simulink model "PosAvail"  (R2018b)
settings: Solver=FixedStepDiscrete  StartTime=0.0  StopTime=10.0  FixedStep=0.01  RelTol=1e-3
settings Model: Creator=su3dcu  LastModifiedBy=su3dcu
settings DataIOCC: SaveFormat=StructureWithTime  ReturnWorkspaceOutputs=on
settings OptimizationCC: DefaultParameterBehavior=Inlined  EnhancedBackFolding=on  PassReuseOutputArgsAs=Individual arguments  ZeroExternalMemoryAtStartup=off  ZeroInternalMemoryAtStartup=off  OptimizeBlockOrder=speed  DifferentSizesBufferReuse=on  OptimizationCustomize=off
settings DebuggingCC: ParameterTunabilityLossMsg=error
settings HardwareCC: ProdBitPerPointer=32  ProdBitPerSizeT=32  ProdBitPerPtrDiffT=32  ProdLargestAtomicFloat=None  ProdWordSize=32  ProdHWDeviceType=Renesas->RH850
settings ModelReferenceCC: ModelReferenceNumInstancesAllowed=Single
settings SFSimCC: SimCustomHeaderCode="#include\"Rte_Type.h\""  MATLABDynamicMemAlloc=off
settings RTWCC: SystemTargetFile=autosar.tlc  GenCodeOnly=on  TemplateMakefile=ert_default_tmf  Description=AUTOSAR  GenerateReport=on  IncludeHyperlinkInReport=on  LaunchReport=on  CodeExecutionProfiling=on  GenerateTraceInfo=on  GenerateTraceReport=on  GenerateTraceReportSl=on  GenerateTraceReportSf=on  GenerateTraceReportEml=on  GenerateCodeMetricsReport=on
settings CodeAppCC: ForceParamTrailComments=on  IgnoreCustomStorageClasses=off  MaxIdLength=63  OperatorAnnotations=on  SimulinkDataObjDesc=on  SFDataObjDesc=on  InsertBlockDesc=on
settings STFCustomTargetCC: TargetLangStandard=C99 (ISO)  MultiwordLength=256  ParMdlRefBuildCompliant=on  CompOptLevelCompliant=on  IncludeMdlTerminateFcn=off  CombineOutputUpdateFcns=on  SuppressErrorStatus=on  ERTCustomFileBanners=on  SupportNonFinite=off  SupportComplex=off  SupportContinuousTime=off  SupportNonInlinedSFcns=off  RemoveResetFunc=on  MATLABClassNameForMDSCustomization=Simulink.SoftwareTarget.ERTCustomization  AutosarCompliant=on  UseToolchainInfoCompliant=on  LookupTableObjectStructAxisOrder=2,1,3,4,...  LUTObjectStructOrderEvenSpacing=Size,Table,Breakpoints  SystemTargetFile=autosar.tlc
settings ERTTargetCC: TargetLangStandard=C99 (ISO)  ConcurrentExecutionCompliant=off  IncludeMdlTerminateFcn=off  SuppressErrorStatus=on  SupportNonFinite=off  SupportComplex=off  ModelStepFunctionPrototypeControlCompliant=off  CPPClassGenCompliant=off  AutosarCompliant=on  LookupTableObjectStructAxisOrder=2,1,3,4,...  LUTObjectStructOrderEvenSpacing=Size,Table,Breakpoints  InlinedParameterPlacement=NonHierarchical  ERTCustomFileTemplate=example_file_process.tlc  ERTFilePackagingFormat=Compact

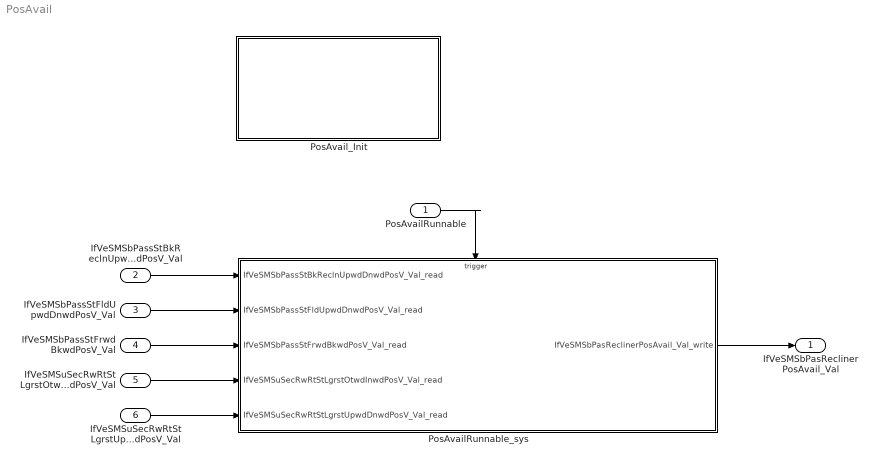
== system PosAvail ==
  PosAvailRunnable : Inport  SampleTime=0.01  OutputFunctionCall=on
  IfVeSMSbPassStBkReclnUpwdDnwdPosV_Val : Inport  Port=2  OutDataTypeStr=boolean  PortDimensions=1
  IfVeSMSbPassStFldUpwdDnwdPosV_Val : Inport  Port=3  OutDataTypeStr=boolean  PortDimensions=1
  IfVeSMSbPassStFrwdBkwdPosV_Val : Inport  Port=4  OutDataTypeStr=boolean  PortDimensions=1
  IfVeSMSuSecRwRtStLgrstOtwdInwdPosV_Val : Inport  Port=5  OutDataTypeStr=boolean  PortDimensions=1
  IfVeSMSuSecRwRtStLgrstUpwdDnwdPosV_Val : Inport  Port=6  OutDataTypeStr=boolean  PortDimensions=1
  PosAvailRunnable_sys : Subsystem
  PosAvail_Init : Subsystem
  IfVeSMSbPasReclinerPosAvail_Val : Outport  OutDataTypeStr=boolean  PortDimensions=1
  wires:
  IfVeSMSbPassStBkReclnUpwdDnwdPosV_Val/1 -> PosAvailRunnable_sys/1(IfVeSMSbPassStBkReclnUpwdDnwdPosV_Val_read)
  IfVeSMSbPassStFldUpwdDnwdPosV_Val/1 -> PosAvailRunnable_sys/2(IfVeSMSbPassStFldUpwdDnwdPosV_Val_read)
  IfVeSMSbPassStFrwdBkwdPosV_Val/1 -> PosAvailRunnable_sys/3(IfVeSMSbPassStFrwdBkwdPosV_Val_read)
  PosAvailRunnable_sys/1(IfVeSMSbPasReclinerPosAvail_Val_write) -> IfVeSMSbPasReclinerPosAvail_Val/1
  PosAvailRunnable/1 -> PosAvailRunnable_sys/Trigger
  IfVeSMSuSecRwRtStLgrstOtwdInwdPosV_Val/1 -> PosAvailRunnable_sys/4(IfVeSMSuSecRwRtStLgrstOtwdInwdPosV_Val_read)
  IfVeSMSuSecRwRtStLgrstUpwdDnwdPosV_Val/1 -> PosAvailRunnable_sys/5(IfVeSMSuSecRwRtStLgrstUpwdDnwdPosV_Val_read)

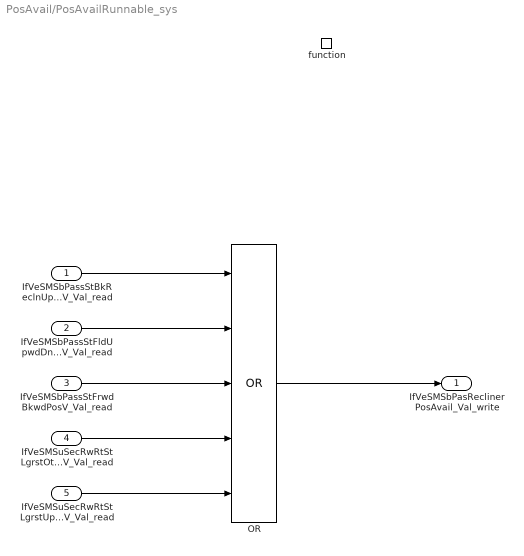
== system PosAvail/PosAvailRunnable_sys ==
  IfVeSMSbPassStBkReclnUpwdDnwdPosV_Val_read : Inport
  IfVeSMSbPassStFldUpwdDnwdPosV_Val_read : Inport  Port=2
  IfVeSMSbPassStFrwdBkwdPosV_Val_read : Inport  Port=3
  IfVeSMSuSecRwRtStLgrstOtwdInwdPosV_Val_read : Inport  Port=4
  IfVeSMSuSecRwRtStLgrstUpwdDnwdPosV_Val_read : Inport  Port=5
  function : TriggerPort  TriggerType=function-call  VariantControl=(inherit)  SampleTimeType=periodic  SampleTime=-1
  OR : Logic  Operator=OR  Inputs=5  AllPortsSameDT=off  OutDataTypeStr=boolean
  IfVeSMSbPasReclinerPosAvail_Val_write : Outport
  wires:
  IfVeSMSbPassStBkReclnUpwdDnwdPosV_Val_read/1 -> OR/1
  IfVeSMSbPassStFldUpwdDnwdPosV_Val_read/1 -> OR/2
  IfVeSMSbPassStFrwdBkwdPosV_Val_read/1 -> OR/3
  OR/1 -> IfVeSMSbPasReclinerPosAvail_Val_write/1
  IfVeSMSuSecRwRtStLgrstOtwdInwdPosV_Val_read/1 -> OR/4
  IfVeSMSuSecRwRtStLgrstUpwdDnwdPosV_Val_read/1 -> OR/5

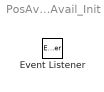
== system PosAvail/PosAvail_Init ==
  Event Listener : EventListener  EventName=reset
